simulink model "MotorPos_Reference"  (R2020b)
settings: Solver=VariableStepAuto  StartTime=0.0  StopTime=10.0  RelTol=1e-3
values from neighbouring files (symbols this model uses):
  b = 3.5077E-6    [IN_Data.sldd]    (also in data.mat = 3.5077e-06)
  J = 3.2284E-6    [IN_Data.sldd]    (also in data.mat = 3.2284e-06)
  K = 0.0274    [IN_Data.sldd]    (also in data.mat)
  L = 2.75E-6    [IN_Data.sldd]    (also in data.mat = 2.75e-06)
  R = 4.0    [IN_Data.sldd]    (also in data.mat = 4)
settings Model: DataDictionary=IN_Data.sldd  Creator=vijay jagtap  LastModifiedBy=vijay jagtap
settings DataIOCC: SaveOutput=off  SaveTime=off

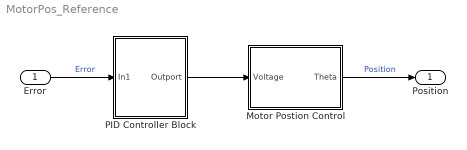
== system MotorPos_Reference ==
  Error : Inport  OutDataTypeStr=double  PortDimensions=1  SampleTime=0
  Motor Postion Control : Subsystem
  PID Controller Block : Subsystem  mask{Kp=17, Ki=423, Kd=0.14, N=3321}
      mask prompts: N "Filter Coefficient"
  Position : Outport  OutDataTypeStr=double  PortDimensions=1  SampleTime=0
  wires:
  PID Controller Block/1(Outport) -> Motor Postion Control/1(Voltage)
  Motor Postion Control/1(Theta) -> Position/1  "Position"
  Error/1 -> PID Controller Block/1(In1)  "Error"

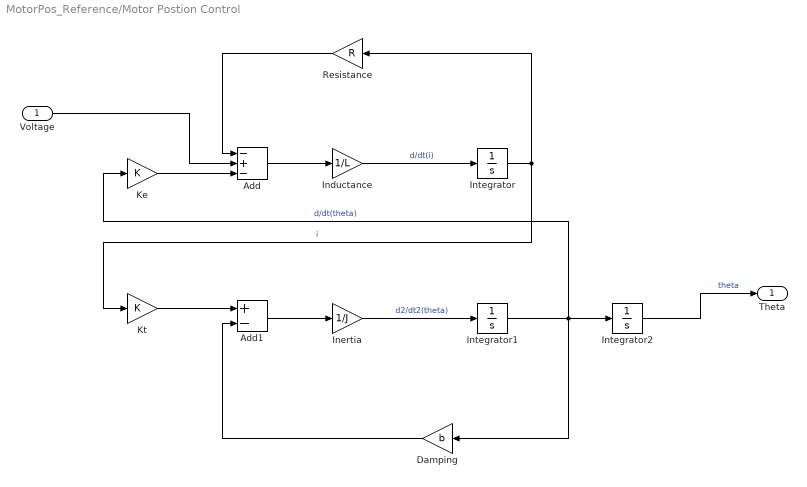
== system MotorPos_Reference/Motor Postion Control ==
  Voltage : Inport
  Add : Sum  Inputs=-+-
  Add1 : Sum  Inputs=+-
  Damping : Gain  Gain=b
  Inductance : Gain  Gain=1/L
  Inertia : Gain  Gain=1/J
  Integrator : Integrator
  Integrator1 : Integrator
  Integrator2 : Integrator
  Ke : Gain  Gain=K
  Kt : Gain  Gain=K
  Resistance : Gain  Gain=R
  Theta : Outport
  wires:
  Integrator2/1 -> Theta/1  "theta"
  Voltage/1 -> Add/2
  Ke/1 -> Add/3
  Resistance/1 -> Add/1
  Damping/1 -> Add1/2
  Inductance/1 -> Integrator/1  "d/dt(i)"
  Kt/1 -> Add1/1
  Integrator/1 -> Resistance/1, Kt/1  "i"
  Add1/1 -> Inertia/1
  Inertia/1 -> Integrator1/1  "d2/dt2(theta)"
  Add/1 -> Inductance/1
  Integrator1/1 -> Integrator2/1, Damping/1, Ke/1  "d/dt(theta)"

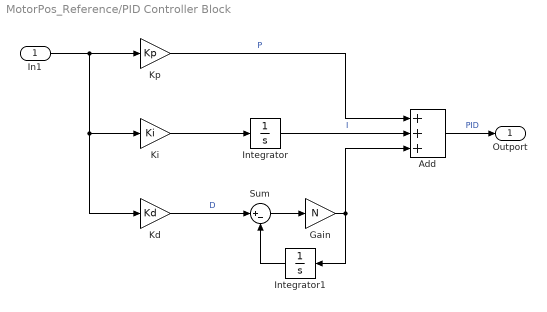
== system MotorPos_Reference/PID Controller Block ==
  In1 : Inport
  Add : Sum  Inputs=+++
  Gain : Gain  Gain=N
  Integrator : Integrator
  Integrator1 : Integrator
  Kd : Gain  Gain=Kd
  Ki : Gain  Gain=Ki
  Kp : Gain  Gain=Kp
  Sum : Sum  Inputs=|+-
  Outport : Outport
  wires:
  Sum/1 -> Gain/1
  Integrator1/1 -> Sum/2
  Gain/1 -> Add/3, Integrator1/1
  Add/1 -> Outport/1  "PID"
  Integrator/1 -> Add/2  "I"
  Kd/1 -> Sum/1  "D"
  Ki/1 -> Integrator/1
  Kp/1 -> Add/1  "P"
  In1/1 -> Kp/1, Ki/1, Kd/1
